simulink model "controlloCoppia_handle_statico"  (R2018b)
settings: Solver=VariableStepAuto  StartTime=0.0  StopTime=1  FixedStep=0.001  RelTol=1e-3
values from neighbouring files (symbols this model uses):
  cond_init = [0, 150/180*pi, pi/3, -pi/2, -3*pi/4,-150/180*pi]'    [init.m]
  Legge = [Kp,Kd]    [LAUNCH_COMP_TORQUE_TRAJ.m]    (also in LAUNCH_PD.m = [Kp Kd]; LAUNCH_PD_TRAJ.m)
  param = param'    [init.m]
settings Model: Creator=Utente  LastModifiedBy=Utente

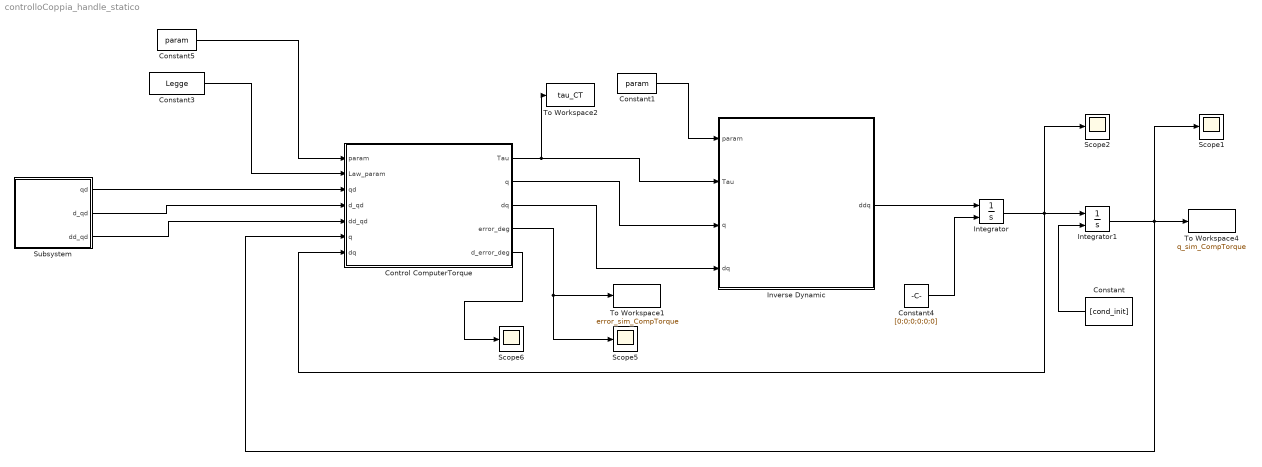
== system controlloCoppia_handle_statico ==
  Constant : Constant  Value=[cond_init]
  Constant1 : Constant  Value=param
  Constant3 : Constant  Value=Legge
  Constant4 : Constant  Value=[0;0;0;0;0;0]
  Constant5 : Constant  Value=param
  Control ComputerTorque : MATLAB Function  TreatAsAtomicUnit=on
  Integrator : Integrator  InitialConditionSource=external  InitialCondition=[0;0;0;0;0;0]
  Integrator1 : Integrator  InitialConditionSource=external
  Inverse Dynamic : MATLAB Function  TreatAsAtomicUnit=on
  Scope{1..2,5..6} (4 alike) : Scope
  Subsystem : Subsystem
  To Workspace1 : ToWorkspace  VariableName=error_sim_CompTorque  SaveFormat=Structure With Time  SampleTime=-1
      settings: Save2DSignal=2-D array (concatenate along first dimension)
  To Workspace2 : ToWorkspace  VariableName=tau_CT  SaveFormat=Structure With Time  SampleTime=-1
      settings: Save2DSignal=2-D array (concatenate along first dimension)
  To Workspace4 : ToWorkspace  VariableName=q_sim_CompTorque  SaveFormat=Structure With Time  SampleTime=-1
      settings: Save2DSignal=2-D array (concatenate along first dimension)
  wires:
  Constant5/1 -> Control ComputerTorque/1(param)
  Constant3/1 -> Control ComputerTorque/2(Law_param)
  Subsystem/1(qd) -> Control ComputerTorque/3(qd)
  Subsystem/2(d_qd) -> Control ComputerTorque/4(d_qd)
  Subsystem/3(dd_qd) -> Control ComputerTorque/5(dd_qd)
  Control ComputerTorque/1(Tau) -> To Workspace2/1, Inverse Dynamic/2(Tau)
  Control ComputerTorque/2(q) -> Inverse Dynamic/3(q)
  Control ComputerTorque/3(dq) -> Inverse Dynamic/4(dq)
  Constant4/1 -> Integrator/2
  Integrator/1 -> Control ComputerTorque/7("dq "), Integrator1/1, Scope2/1
  Integrator1/1 -> Control ComputerTorque/6("q "), To Workspace4/1, Scope1/1
  Inverse Dynamic/1(ddq) -> Integrator/1
  Constant/1 -> Integrator1/2
  Constant1/1 -> Inverse Dynamic/1(param)
  Control ComputerTorque/4(error_deg) -> Scope5/1, To Workspace1/1
  Control ComputerTorque/5(d_error_deg) -> Scope6/1

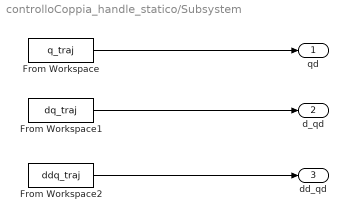
== system controlloCoppia_handle_statico/Subsystem ==
  From Workspace : FromWorkspace  VariableName=q_traj  SampleTime=0
  From Workspace1 : FromWorkspace  VariableName=dq_traj  SampleTime=0
  From Workspace2 : FromWorkspace  VariableName=ddq_traj  SampleTime=0
  qd : Outport
  d_qd : Outport  Port=2
  dd_qd : Outport  Port=3
  wires:
  From Workspace/1 -> qd/1
  From Workspace1/1 -> d_qd/1
  From Workspace2/1 -> dd_qd/1

== matlab function controlloCoppia_handle_statico/Control ComputerTorque ==
  data: param input; Tau output; Law_param input; qd input; d_qd input; dd_qd input; q input; dq input; q output; dq output; error_deg output; d_error_deg output
function [Tau,q,dq,error_deg,d_error_deg] = ComputerTorqueControl(param, Law_param,  qd, d_qd, dd_qd,  q,dq)

    I = eye(size(q,1));

    Kp = Law_param(1)*I;
    Kd = Law_param(2)*I;

    [B,C,G] = Dinamica_new(param,q,dq);
    error = (qd-q);
    d_error = (d_qd-dq);
    
    error_deg = 180/pi*(qd-q);
    d_error_deg = 180/pi*(d_qd-dq);
        
    Tau = B*dd_qd + Kp*error + Kd*d_error + C*dq + G;
    
    
end

== matlab function controlloCoppia_handle_statico/Inverse Dynamic ==
  data: param input; Tau input; ddq output; q input; dq input
function ddq = inverseD(param,Tau,q,dq)

    [B,C,G] = Dinamica_new(param,q,dq);
    tot = Tau - C*dq - G;
    
    ddq = B\(tot);
    
end
